simulink model "motore_regolato"  (Simulink 7.7)
settings: Solver=ode45  StartTime=0.0  StopTime=2.0  RelTol=1e-9  AbsTol=1e-9
values from neighbouring files (symbols this model uses):
  Atilde = [-h/J 0; -1 0]    [motore.m]    (also in produzione.m = [0 (1-alpha)*(1-beta2) 0; 1-beta1 0 0; 0 -alpha*(1-beta2) 1])
  btilde = [nu/J; 0]    [motore.m]    (also in produzione.m = [1; 0; 0])
  ctilde = [0 1]    [motore.m]    (also in produzione.m = [0 0 1])
  dist = -3    [motore.m]    (also in produzione.m = 3)
  h = 200    [antenna.m]    (also in motore.m = 20)
  J = 1500    [antenna.m]    (also in motore.m = 1)
  k = [k1 k2]    [antenna.m]    (also in motore.m; produzione.m = [k1 k2 k3]; serbatoi.m)
  l = [l1; l2]    [antenna.m]    (also in motore.m; produzione.m = [l1; l2; l3]; serbatoi.m)
  nu = 100    [motore.m]
  y0 = 0.5    [antenna.m]    (also in motore.m = 5; produzione.m = 50; serbatoi.m = 5)
settings Model: Creator=fabio  LastModifiedBy=fabio

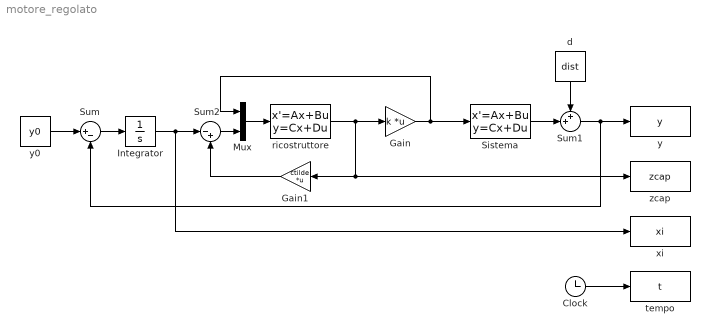
== system motore_regolato ==
  Clock : Clock
      settings: Decimation=10
  Gain : Gain  Gain=k  Multiplication=Matrix(K*u)
  Gain1 : Gain  Gain=ctilde  Multiplication=Matrix(K*u)
  Integrator : Integrator
  Mux : Mux  Inputs=2
  Sistema : StateSpace  A=-h/J  B=nu/J  D=0
  Sum : Sum  Inputs=|+-
  Sum1 : Sum  Inputs=++|
  Sum2 : Sum  Inputs=|-+
  d : Constant  Value=dist
  ricostruttore : StateSpace  A=Atilde  B=[btilde l]  C=[1 0; 0 1]  D=[0 0; 0 0]  X0=[0 0]'
  tempo : ToWorkspace  VariableName=t  SampleTime=-1  SaveFormat=Array
  xi : ToWorkspace  VariableName=xi  SampleTime=-1  SaveFormat=Array
  y : ToWorkspace  VariableName=y  SampleTime=-1  SaveFormat=Array
  y0 : Constant  Value=y0
  zcap : ToWorkspace  VariableName=zcap  SampleTime=-1  SaveFormat=Array
  wires:
  y0/1 -> Sum/1
  Sum/1 -> Integrator/1
  ricostruttore/1 -> Gain/1, zcap/1, Gain1/1
  Gain/1 -> Mux/1, Sistema/1
  Mux/1 -> ricostruttore/1
  Clock/1 -> tempo/1
  Gain1/1 -> Sum2/2
  Integrator/1 -> Sum2/1, xi/1
  Sum2/1 -> Mux/2
  d/1 -> Sum1/1
  Sum1/1 -> y/1, Sum/2
  Sistema/1 -> Sum1/2
